simulink model "model"  (R2021a)
settings: Solver=VariableStepAuto  StartTime=0.0  StopTime=10.0  RelTol=1e-3
values from neighbouring files (symbols this model uses):
  p_0 = -2.9998e-06    [main.m]    (also in main_params_plot.m = 1; measure.m = 1)
  p_1 = 0.32977    [main.m]    (also in main_params_plot.m = 1; measure.m = 1)
  p_2 = -0.0054782    [main.m]    (also in main_params_plot.m = 1; measure.m = 1)
  p_3 = -0.0022903    [main.m]    (also in main_params_plot.m = 1; measure.m = 1)
  p_4 = 0.033036    [main.m]
settings Model: OrderedModelArguments=off  Creator=artem  LastModifiedBy=artof
settings SolverCC: AlgebraicLoopSolver=TrustRegion
settings DebuggingCC: SFMachineParentedDataDiag=warning

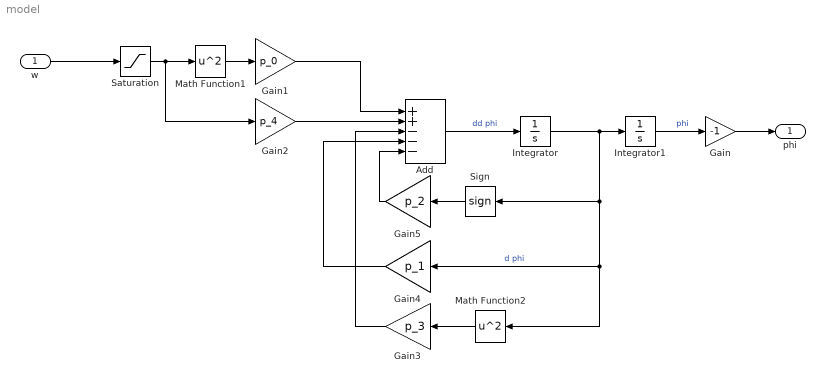
== system model ==
  w : Inport
  Add : Sum  Inputs=++---
  Gain : Gain  Gain=-1
  Gain1 : Gain  Gain=p_0
  Gain2 : Gain  Gain=p_4
  Gain3 : Gain  Gain=p_3
  Gain4 : Gain  Gain=p_1
  Gain5 : Gain  Gain=p_2
  Integrator : Integrator  ZeroCross=off
  Integrator1 : Integrator  ZeroCross=off
  Math Function1 : Math  Operator=square  SaturateOnIntegerOverflow=on
  Math Function2 : Math  Operator=square  SaturateOnIntegerOverflow=on
  Saturation : Saturate  UpperLimit=125  LowerLimit=-125
  Sign : Signum
  phi : Outport
  wires:
  Math Function2/1 -> Gain3/1
  w/1 -> Saturation/1
  Gain3/1 -> Add/3
  Gain2/1 -> Add/2
  Gain1/1 -> Add/1
  Integrator/1 -> Integrator1/1, Math Function2/1, Gain4/1, Sign/1  "d phi"
  Sign/1 -> Gain5/1
  Gain4/1 -> Add/4
  Integrator1/1 -> Gain/1  "phi"
  Saturation/1 -> Gain2/1, Math Function1/1
  Gain5/1 -> Add/5
  Gain/1 -> phi/1
  Add/1 -> Integrator/1  "dd phi"
  Math Function1/1 -> Gain1/1
